simulink model "IKTrajectoryControlExample"  (R2019b)
settings: Solver=ode3  StartTime=0.0  StopTime=40  FixedStep=Ts  RelTol=1e-3
PostLoadFcn:
  | sawyer = importrobot('sawyer.urdf');
  | sawyer.DataFormat = 'column';
  | 
  | I = imread('coins.png');
  | imageOrigin = [0.4,0.2,0.08];
  | scale = .0015;
model workspace (MAT data in the model file):
  I = [49 47 48 48 48 48 48 51 50 51 50 47 ... (73800 elements, 246x300)]
  Ts = 0.01
  filterConst = 0.08
  force_range = [0.8 0.9]
  imageOrigin = [0.4 0.2 0.08]
  initTargetPose = [-1 0 -1.22464679915e-16 0 0 1 0 0 1.22464679915e-16 0 -1 0 ... (16 elements, 4x4)]
  q0 = [0.422405030154; 0; -1.22880122285; -0.410622115963; 2.12106389539; 0.205505693545; 0.715545053124; 1.62245603969]
  robot : robotics.RigidBodyTree (value not decoded)
  sawyer : robotics.RigidBodyTree (value not decoded)
  scale = 0.0015
  wayPoints = [0.4 0.4 0.4 0.4 0.4 0.4 0.4 0.4 0.4 0.4 0.4 0.4 ... (9846 elements, 1641x6)]
  weights = [1 1 1 1 1 1]
  weights1 = [1 1 1 1 1 1]
undefined symbols (not defined in the file or in its folder): Levenberg, Marquardt
libraries: robotmaniplib x6, simulink x5, robotcorelib x1
(part 2 of 2)

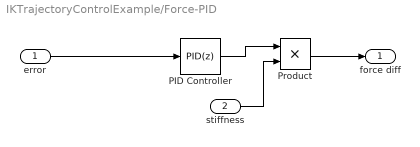
== system IKTrajectoryControlExample/Force-PID ==
  error : Inport
  stiffness : Inport  Port=2
  PID Controller : simulink/Continuous/PID Controller  Controller=PID  Form=Parallel  TimeDomain=Discrete-time  SampleTime=0.01  IntegratorMethod=Forward Euler  FilterMethod=Forward Euler  ControllerParametersSource=internal  P=0.03  I=0.3  D=10  UseFilter=on  N=0  TunerSelectOption=Transfer Function Based (PID Tuner App)  InitialConditionSource=internal  InitialConditionForIntegrator=0  InitialConditionForFilter=0  DifferentiatorICPrevScaledInput=0  ExternalReset=none  TrackingMode=off  Kt=1  LimitOutput=off  UpperSaturationLimit=inf  LowerSaturationLimit=-inf  LinearizeAsGain=on  AntiWindupMode=none  Kb=1  POutMin=[]  POutMax=[]  IOutMin=[]  IOutMax=[]  DOutMin=[]  DOutMax=[]  NOutMin=[]  NOutMax=[]  SumOutMin=[]  SumOutMax=[]  SaturationOutMin=[]  SaturationOutMax=[]  PParamMin=[]  PParamMax=[]  IParamMin=[]  IParamMax=[]  DParamMin=[]  DParamMax=[]  NParamMin=[]  NParamMax=[]  KbParamMin=[]  KbParamMax=[]  KtParamMin=[]  KtParamMax=[]  KbOutMin=[]  KbOutMax=[]  KtOutMin=[]  KtOutMax=[]  IntegratorOutMin=[]  IntegratorOutMax=[]  FilterOutMin=[]  FilterOutMax=[]  SumI1OutMin=[]  SumI1OutMax=[]  SumI2OutMin=[]  SumI2OutMax=[]  SumI3OutMin=[]  SumI3OutMax=[]  SumI4OutMin=[]  SumI4OutMax=[]  SumDOutMin=[]  SumDOutMax=[]  DifferentiatorOutMin=[]  DifferentiatorOutMax=[]  FilterDiffOutCoefMin=[]  FilterDiffOutCoefMax=[]  ReciprocalOutMin=[]  ReciprocalOutMax=[]  SumDenOutMin=[]  SumDenOutMax=[]  SumNumOutMin=[]  SumNumOutMax=[]  DivideOutMin=[]  DivideOutMax=[]  IntegratorContinuousStateAttributes=''  IntegratorStateMustResolveToSignalObject=off  IntegratorRTWStateStorageClass=Auto  FilterContinuousStateAttributes=''  FilterStateMustResolveToSignalObject=off  FilterRTWStateStorageClass=Auto  ParallelPVariant=InternalParameters  IdealPVariant=Disabled  IVariant=InternalParameters  DVariant=InternalParameters  IntegratorVariant=Discrete  SatVariant=Disabled  AWVariant=Passthrough  PCopyVariant=Disabled  TRVariant=Disabled  FdbkBlocksVariant=Forward  IdealPFdbkVariant=Disabled  SatFdbkVariant=Disabled  DerivativeFilterVariant=ForwardEulerFilter  NVariant=InternalParameters  NCopyVariant=Disabled  FilterICVariant=InternalICsFilter  IntegratorICVariant=InternalICs  ExternalResetVariant=Disabled  TRSumVariant=Passthrough  SumFdbkVariant=Disabled  SumVariant=Sum_PID
  Product : Product
  force diff : Outport
  wires:
  error/1 -> PID Controller/1
  PID Controller/1 -> Product/1
  stiffness/1 -> Product/2
  Product/1 -> force diff/1

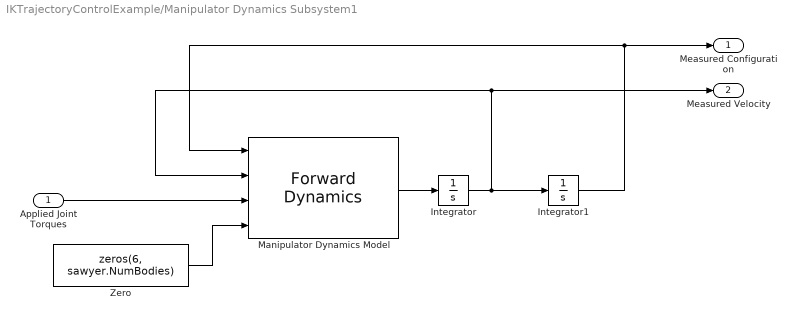
== system IKTrajectoryControlExample/Manipulator Dynamics Subsystem1 ==
  Applied Joint Torques : Inport
  Integrator : Integrator
  Integrator1 : Integrator  InitialCondition=q0
  Manipulator Dynamics Model : robotmaniplib/Forward Dynamics  RigidBodyTree=sawyer  SimulateUsing=Interpreted execution
      settings: SourceProductName=Robotics System Toolbox
  Zero : Constant  Value=zeros(6, sawyer.NumBodies)  OutDataTypeStr=Inherit: Inherit via back propagation
  Measured Configuration : Outport  VectorParamsAs1DForOutWhenUnconnected=off
  Measured Velocity : Outport  Port=2  VectorParamsAs1DForOutWhenUnconnected=off
  wires:
  Integrator1/1 -> Manipulator Dynamics Model/1, Measured Configuration/1
  Manipulator Dynamics Model/1 -> Integrator/1
  Integrator/1 -> Integrator1/1, Manipulator Dynamics Model/2, Measured Velocity/1
  Applied Joint Torques/1 -> Manipulator Dynamics Model/3
  Zero/1 -> Manipulator Dynamics Model/4

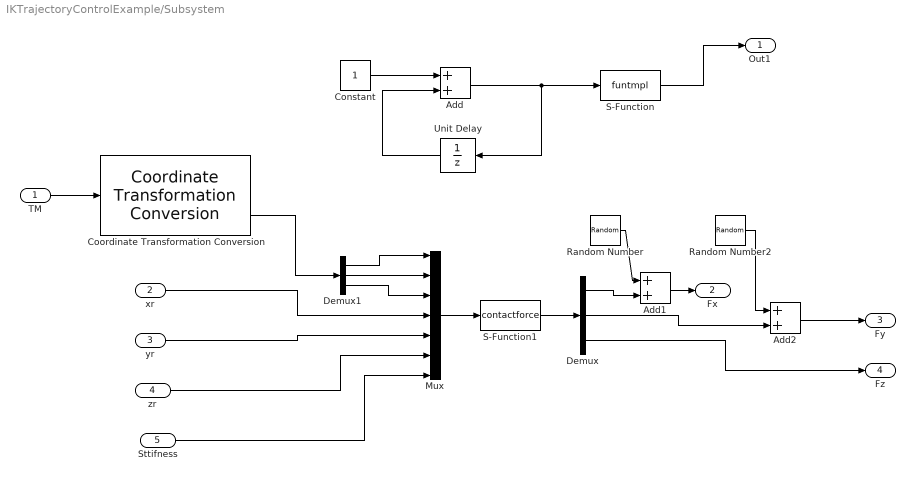
== system IKTrajectoryControlExample/Subsystem ==
  TM : Inport
  xr : Inport  Port=2
  yr : Inport  Port=3
  zr : Inport  Port=4
  "Sttifness " : Inport  Port=5
  Add : Sum
  Add1 : Sum
  Add2 : Sum
  Constant : Constant
  Coordinate Transformation Conversion : robotcorelib/Coordinate Transformation Conversion  InputRepresentation=Homogeneous Transformation  InputEulerSequence=ZYX  ShowTrVecInputPort=on  OutputRepresentation=Rotation Matrix  OutputEulerSequence=ZYX  ShowTrVecOutputPort=on  SimulateUsing=Interpreted execution
      settings: SourceProductBaseCode=RO
  Demux : Demux  Outputs=3
  Demux1 : Demux  Outputs=3
  Mux : Mux  Inputs=7
  Random Number : RandomNumber  Variance=0.001  SampleTime=0.01
  Random Number2 : RandomNumber  Variance=0.001  SampleTime=0.01
  S-Function : S-Function  FunctionName=funtmpl  SFunctionDeploymentMode=off  EnableBusSupport=off
  S-Function1 : S-Function  FunctionName=contactforce  SFunctionDeploymentMode=off  EnableBusSupport=off
  Unit Delay : UnitDelay  SampleTime=-1  HasFrameUpgradeWarning=on
  Out1 : Outport
  Fx : Outport  Port=2
  Fy : Outport  Port=3
  Fz : Outport  Port=4
  wires:
  S-Function/1 -> Out1/1
  Constant/1 -> Add/1
  Add/1 -> Unit Delay/1, S-Function/1
  Unit Delay/1 -> Add/2
  TM/1 -> Coordinate Transformation Conversion/1
  xr/1 -> Mux/4
  yr/1 -> Mux/5
  zr/1 -> Mux/6
  Mux/1 -> S-Function1/1
  S-Function1/1 -> Demux/1
  Add1/1 -> Fx/1
  Demux/1 -> Add1/2
  Random Number/1 -> Add1/1
  Add2/1 -> Fy/1
  Random Number2/1 -> Add2/1
  Demux/2 -> Add2/2
  "Sttifness "/1 -> Mux/7
  Coordinate Transformation Conversion/2 -> Demux1/1
  Demux1/1 -> Mux/1
  Demux1/2 -> Mux/2
  Demux1/3 -> Mux/3
  Demux/3 -> Fz/1

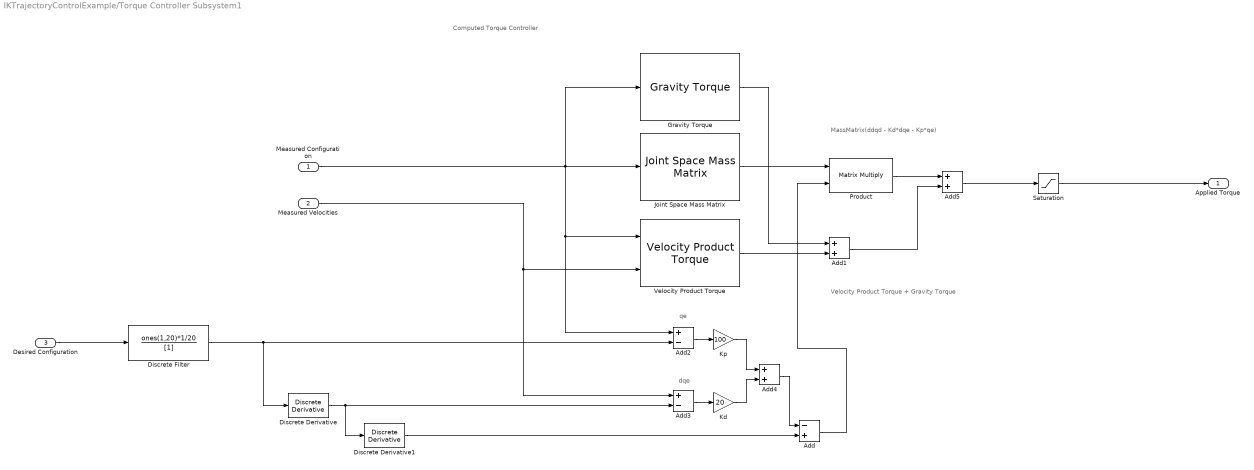
== system IKTrajectoryControlExample/Torque Controller Subsystem1 ==
  note: Computed Torque Controller
  note: MassMatrix(ddqd - Kd*dqe - Kp*qe)
  note: Velocity Product Torque + Gravity Torque
  note: dqe
  note: qe
  Measured Configuration : Inport
  Measured Velocities : Inport  Port=2
  Desired Configuration : Inport  Port=3
  Add : Sum  Inputs=-+
  Add1 : Sum
  Add2 : Sum  Inputs=+-
  Add3 : Sum  Inputs=+-
  Add4 : Sum
  Add5 : Sum
  Discrete Derivative : simulink/Discrete/Discrete Derivative  gainval=1.0  ICPrevScaledInput=0.0  OutMin=[]  OutMax=[]  OutDataType=fixdt(1, 16)  OutScaling=2^-10  DoSatur=off
  Discrete Derivative1 : simulink/Discrete/Discrete Derivative  gainval=1.0  ICPrevScaledInput=0.0  OutMin=[]  OutMax=[]  OutDataType=fixdt(1, 16)  OutScaling=2^-10  DoSatur=off
  Discrete Filter : DiscreteFilter  Numerator=ones(1,20)*1/20  Denominator=[1]  InitialStates=repmat(q0',19,1)
  Gravity Torque : robotmaniplib/Gravity Torque  RigidBodyTree=sawyer  SimulateUsing=Interpreted execution
      settings: SourceProductName=Robotics System Toolbox
  Joint Space Mass Matrix : robotmaniplib/Joint Space Mass Matrix  RigidBodyTree=sawyer  SimulateUsing=Interpreted execution
      settings: SourceProductName=Robotics System Toolbox
  Kd : Gain  Gain=20
  Kp : Gain  Gain=100
  Product : Product  Multiplication=Matrix(*)
  Saturation : Saturate  UpperLimit=100  LowerLimit=-100
  Velocity Product Torque : robotmaniplib/Velocity Product Torque  RigidBodyTree=sawyer  SimulateUsing=Interpreted execution
      settings: SourceProductName=Robotics System Toolbox  SourceProductBaseCode=RO
  Applied Torque : Outport  VectorParamsAs1DForOutWhenUnconnected=off
  wires:
  Saturation/1 -> Applied Torque/1
  Velocity Product Torque/1 -> Add1/2
  Gravity Torque/1 -> Add1/1
  Add1/1 -> Add5/2
  Product/1 -> Add5/1
  Add5/1 -> Saturation/1
  Kd/1 -> Add4/2
  Kp/1 -> Add4/1
  Add3/1 -> Kd/1
  Add2/1 -> Kp/1
  Discrete Derivative/1 -> Add3/2, Discrete Derivative1/1
  Desired Configuration/1 -> Discrete Filter/1
  Add/1 -> Product/2
  Discrete Derivative1/1 -> Add/2
  Add4/1 -> Add/1
  Measured Velocities/1 -> Velocity Product Torque/2, Add3/1
  Measured Configuration/1 -> Add2/1, Velocity Product Torque/1, Gravity Torque/1, Joint Space Mass Matrix/1
  Joint Space Mass Matrix/1 -> Product/1
  Discrete Filter/1 -> Discrete Derivative/1, Add2/2

== stateflow chart IKTrajectoryControlExample/Waypoint Selection//Conversion Logic1 ==
  (default) -> (junction 1) : %Check EE deviation from Target Pose
      | {error = vecnorm(targetPose(1:3, :) - currentEEPose(1:3, :), 2, 1); }
  (junction 1) -> (junction 3) [order 1] : [(Stop_Force_Control==true &&  all(error < tol ))]
  (junction 3) -> (junction 19) [order 1] : [index == length(wayPoints)]
  (junction 1) -> (junction 5) [order 2]
  (junction 3) -> (junction 7) [order 2] : %Select next Waypoint
      | {index = index + 1;
      | }
  (junction 19) -> (junction 22) : %Stop Simulation
      | {finished = true;}
  (junction 7) -> (junction 5)
  (junction 22) -> (junction 7)
  (junction 5) -> (junction 10) : %Update Target and Convert to Homogenous Transform disp(targetPose);
      | { targetPose = eul2tform(wayPoints(index,4:6));
      | targetPose(1:3,end) = (wayPoints(index,1:3)+[0 0 force_diff])';
      | }
  data: targetPose output =initTargetPose; wayPoints input; currentEEPose input; finished output =false; index local [..length(wayPoints)] =1; tol local =.01; error local; Stop_Force_Control input; force_diff input

== matlab function IKTrajectoryControlExample/MATLAB Function1 ==
  data: targetPose input; wayPoints input; currentPose input
function waypointTracking(targetPose, wayPoints, currentPose)
%#codegen

persistent f1 a1

if isempty(f1)
    f1 = figure;
    title('Waypoint Tracking-force');
    a1 = axes;
    axis(a1, [	0.4,0.8, 0.2,0.635, 0.05,0.3]);
    set(f1, 'Visible', 'on');
end

targetPoint = targetPose(1:3,end);
currentPoint = currentPose(1:3,end);

plot3(a1,wayPoints(:,1), wayPoints(:,2), wayPoints(:,3), 'b.', 'MarkerSize', 1);
hold on
plot3(a1,targetPoint(1), targetPoint(2), targetPoint(3), 'go', 'MarkerSize', 5);
plot3(a1,currentPoint(1), currentPoint(2), currentPoint(3), 'ro', 'MarkerSize', 5);

hold off
